simulink model "Example_3"  (R2020b)
settings: Solver=VariableStepAuto  StartTime=0.0  StopTime=2  RelTol=1e-3
libraries: fl_lib x8, nesl_utility x4, slctrlblks x1, simulink x1, ee_lib x1
settings Model: Creator=zaliyazici  LastModifiedBy=zaliyazici

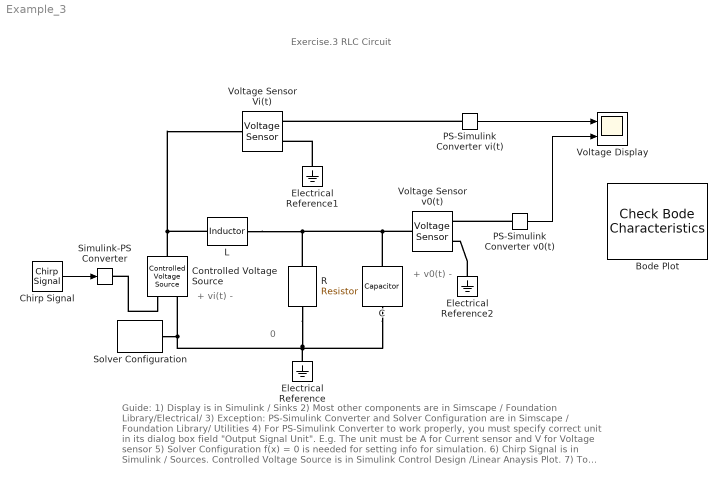
== system Example_3 ==
  note: Exercise.3 RLC Circuit
  note: 0
  note: +
      | v0(t)
      | -
  note: +
      | vi(t)
      | -
  note: Guide:
      | 1) Display is in Simulink / Sinks
      | 2) Most other components are in Simscape / Foundation Library/Electrical/
      | 3) Exception: PS-Simulink Converter and Solver Configuration are in Simscape / Foundation Library/ Utilities
      | 4) For PS-Simulink Converter to work properly, you must specify correct unit in its dialog box field "Output Signal Unit".
      | E.g. The unit must be A for Current sensor and V for Voltage sensor
      | 5) Solver Configuration f(x) = 0 is needed for setting info for simulation.
      | 6) Chirp Signal is in Simulink / Sources. Controlled Voltage Source is in Simulink Control Design /Linear Anaysis Plot.
      | 7) To create "Annotation", double-click a location on project page and select "Create annotation" from the prompt. Then, type any text you want to clarify your circuit. E.g. "Display for Voltage".
      | 8) To understand how to use a component, right-click on the component and select "Help".
      | Measurement: $V_i(\omega), V_0(\omega)$
  Bode Plot : slctrlblks/Model Verification/Check Bode  Characteristics  InstantiateOnLoad=on  SaveOperatingPoints=off  LinearizationIOs={'/Chirp Signal', 1, 'in', 'off', '';'/PS-Simulink Converter v0(t)', 1, 'out', 'off', ''}  LinearizeAt=SnapshotTimes  SnapshotTimes=[0]  TriggerType=rising  SampleTime=auto  RateConversionMethod=zoh  PreWarpFreq=10  UseExactDelayModel=off  UseFullBlockNameLabels=off  UseBusSignalLabels=off  enabled=on  stopWhenAssertionFail=off  export=off  ViewDlgPos=[2923 314 809 588]  OpenViewOnLoad=on  LaunchViewOnOpen=on  FrequencyUnits=rad/s  MagnitudeUnits=dB  PhaseUnits=deg  TimeUnits=seconds  EnableUpperBound=off  UpperBoundFrequencies=[]  UpperBoundMagnitudes=[]  EnableLowerBound=off  LowerBoundFrequencies=[]  LowerBoundMagnitudes=[]
      settings: SaveToWorkspace=on
  C : fl_lib/Electrical/Electrical Elements/Capacitor  c=0.01 uF  r=1e-6 Ohm  g=0 1/Ohm  i_specify=off  i_priority=None  i=0 A  i_nominal_specify=off  i_nominal_unit=A  i_nominal_value=1  v_specify=off  v_priority=None  v=0 V  v_nominal_specify=off  v_nominal_unit=V  v_nominal_value=1  vc_specify=on  vc_priority=High  vc=0 V  vc_nominal_specify=off  vc_nominal_unit=V  vc_nominal_value=1
      settings: AttributesFormatString=%<c> %<c_unit>
  Chirp Signal : simulink/Sources/Chirp Signal  f1=10  T=10  f2=10000
  Controlled Voltage Source : fl_lib/Electrical/Electrical Sources/Controlled Voltage Source
  Electrical Reference : fl_lib/Electrical/Electrical Elements/Electrical Reference
  Electrical Reference1 : fl_lib/Electrical/Electrical Elements/Electrical Reference
  Electrical Reference2 : fl_lib/Electrical/Electrical Elements/Electrical Reference
  L : fl_lib/Electrical/Electrical Elements/Inductor  l=40 mH  r=0 Ohm  g=1e-9 1/Ohm  i_specify=off  i_priority=None  i=0 A  i_nominal_specify=off  i_nominal_unit=A  i_nominal_value=1  v_specify=off  v_priority=None  v=0 V  v_nominal_specify=off  v_nominal_unit=V  v_nominal_value=1  i_L_specify=on  i_L_priority=High  i_L=0 mA  i_L_nominal_specify=off  i_L_nominal_unit=A  i_L_nominal_value=1
      settings: AttributesFormatString=%<l> %<l_unit>
  PS-Simulink Converter v0(t) : nesl_utility/PS-Simulink Converter  PhysicalDomain=network_engine_domain  SubClassName=ps_output  LeftPortType=input  RightPortType=output  PseudoPeriodic=off  Frequencies=[]  Unit=V  AffineConversion=off
  PS-Simulink Converter vi(t) : nesl_utility/PS-Simulink Converter  PhysicalDomain=network_engine_domain  SubClassName=ps_output  LeftPortType=input  RightPortType=output  PseudoPeriodic=off  Frequencies=[]  Unit=V  AffineConversion=off
  R : ee_lib/Passive/Resistor  R=2 kOhm  R_tol=5  enable_R_tol=0  tol_distribution=1  nSigma=4  enable_operating_limits=0  operating_limit_action=2  max_working_voltage=100 V  power_rating=1 W  enable_faults=0  fault_action=1  R_faulted=inf Ohm  enable_temporal_fault=0  t_fault=1 s  enable_behavioral_fault=0  max_permissible_current=1 A  t_fail_on_current=1 s  noise_mode=0  sample_time=1e-3 s  repeatability=1  auto_seed=595387449  user_seed=0  Tdevice=25 degC  alpha=3.93e-3 1/K  Tmeas=25 degC  thermal_mass=100 J/K  power_derating_T1=70 degC  power_derating_T2=155 degC  operating_temperature_range_vec=[-50, 150] degC  temperature_specify=off  temperature_priority=High  temperature=298.15 K  temperature_nominal_specify=off  temperature_nominal_unit=K  temperature_nominal_value=1
      settings: AttributesFormatString=%<R> %<R_unit>
  Simulink-PS Converter : nesl_utility/Simulink-PS Converter  PhysicalDomain=network_engine_domain  SubClassName=ps_input  LeftPortType=input  RightPortType=output  PseudoPeriodic=off  Frequencies=[]  NoiseDistribution=none  NoiseParameters=[]  Unit=1  AffineConversion=off  FilteringAndDerivatives=provide  SimscapeFilterOrder=1  InputFilterTimeConstant=0.001  UdotUserProvided=0
  Solver Configuration : nesl_utility/Solver Configuration  PhysicalDomain=network_engine_domain  SubClassName=solver  LeftPortType=input  RightPortType=generic  Tones=[]  Harmonics=[]  SimulateNoise=off  Profile=off  UseLocalSampling=off  EnableSwitchedLinearOptims=on  FrequencyDomain=off  UseCCode=off  RelTol=0.001  AbsTol=1e-06  MinStep=1e-09  ToWorkspace=off  RevertToSquareIcSolve=off  NumHomotopyIterations=100  PhasorMode=off  PhasorModeNumHarmonics=1  DoDC=off  ResidualTolerance=1e-09  UseLocalSolver=off  LocalSolverChoice=NE_BACKWARD_EULER_ADVANCER  LocalSolverSampleTime=0.001  DoFixedCost=off  MaxNonlinIter=3  MaxModeIter=2  ComputeImpulses=off  ImpulseIterations=2  LinearAlgebra=auto  EquationFormulation=NE_TIME_EF  DelaysMemoryBudget=1024  AutomaticFiltering=on  FilteringTimeConstant=0.001  PartitionStorageMethod=AS_NEEDED  PartitionMemoryBudget=1024  PartitionMethod=ROBUST
  Voltage Display : Scope  NumInputPorts=2
  Voltage Sensor Vi(t) : fl_lib/Electrical/Electrical Sensors/Voltage Sensor
  Voltage Sensor v0(t) : fl_lib/Electrical/Electrical Sensors/Voltage Sensor
  wires:
  PS-Simulink Converter v0(t)/1 -> Voltage Display/2
  PS-Simulink Converter vi(t)/1 -> Voltage Display/1
  Chirp Signal/1 -> Simulink-PS Converter/1
  connections:
  PS-Simulink Converter v0(t)/LConn1 -- Voltage Sensor v0(t)/RConn1
  Voltage Sensor v0(t)/LConn1 -- L/RConn1 -- R/LConn1 -- C/LConn1
  Controlled Voltage Source/LConn1 -- L/LConn1 -- Voltage Sensor Vi(t)/LConn1
  PS-Simulink Converter vi(t)/LConn1 -- Voltage Sensor Vi(t)/RConn1
  Controlled Voltage Source/RConn1 -- Simulink-PS Converter/RConn1
  Electrical Reference/LConn1 -- R/RConn1 -- Solver Configuration/RConn1 -- Controlled Voltage Source/RConn2 -- C/RConn1
  Electrical Reference1/LConn1 -- Voltage Sensor Vi(t)/RConn2
  Electrical Reference2/LConn1 -- Voltage Sensor v0(t)/RConn2
